simulink model "smc"  (R2018a)
settings: Solver=VariableStepAuto  StartTime=0.0  StopTime=500  RelTol=1e-3
values from neighbouring files (symbols this model uses):
  D = 0    [k_func.m]
libraries: simulink_extras x5, dspmtrx3 x3, sharedutil x3
settings Model: Creator=Renz  LastModifiedBy=Renz

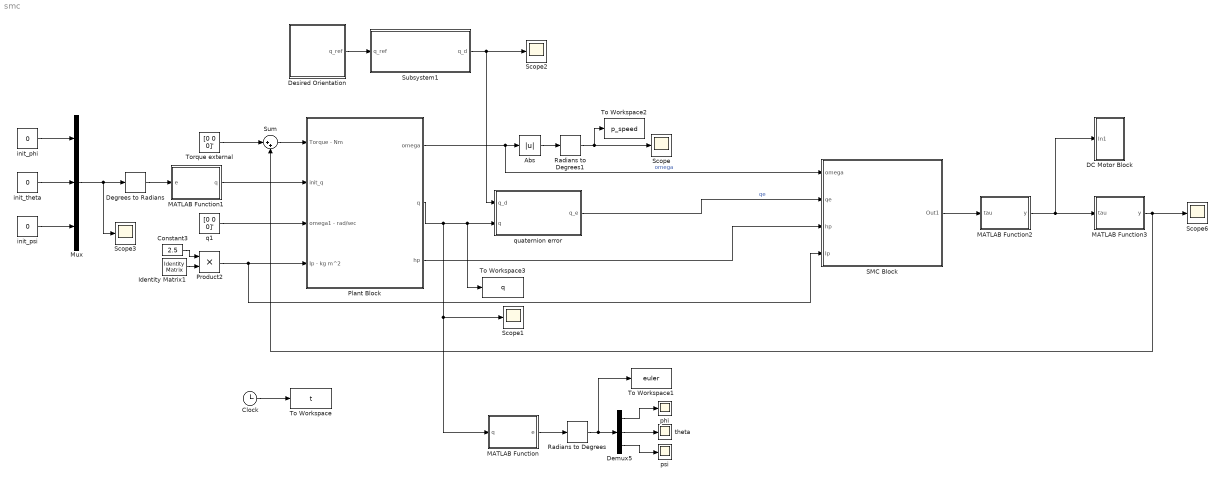
== system smc ==
  Abs : Abs
  Clock : Clock
  Constant3 : Constant  Value=2.5
  DC Motor Block : Subsystem
  Degrees to Radians : simulink_extras/Transformations/Degrees to Radians
  Demux5 : Demux  Outputs=3
  Desired Orientation : Subsystem
  Identity Matrix1 : dspmtrx3/Identity Matrix  Inherit=off  N=3  Ts=1  dataType=double  isSigned=on  wordLen=16  udDataType=sfix(16)  fracBitsMode=Best precision  numFracBits=15  OutDataTypeStr=double  LastOutDataTypeStr=double
      settings: SourceProductName=DSP System Toolbox
  MATLAB Function : MATLAB Function  TreatAsAtomicUnit=on
  MATLAB Function1 : MATLAB Function  TreatAsAtomicUnit=on
  MATLAB Function2 : MATLAB Function  TreatAsAtomicUnit=on
  MATLAB Function3 : MATLAB Function  TreatAsAtomicUnit=on
  Mux : Mux  Inputs=3
  Plant Block : Subsystem
  Product2 : Product
  Radians to Degrees : simulink_extras/Transformations/Radians to Degrees
  Radians to Degrees1 : simulink_extras/Transformations/Radians to Degrees
  SMC Block : Subsystem
  Scope{,1..3,6} (5 alike) : Scope
  Subsystem1 : Subsystem
  Sum : Sum  Inputs=|++
  To Workspace : ToWorkspace  VariableName=t  SampleTime=-1
  To Workspace1 : ToWorkspace  VariableName=euler  SampleTime=-1
  To Workspace2 : ToWorkspace  VariableName=p_speed  SampleTime=-1
  To Workspace3 : ToWorkspace  VariableName=q  SampleTime=-1
  Torque external : Constant  Value=[0 0 0]'
  init_phi : Constant  Value=0
  init_psi : Constant  Value=0
  init_theta : Constant  Value=0
  phi : Scope
  psi : Scope
  q1 : Constant  Value=[0 0 0]'
  quaternion error : Subsystem
  theta : Scope
  wires:
  Identity Matrix1/1 -> Product2/2
  MATLAB Function1/1(q) -> Plant Block/2(init_q)
  Torque external/1 -> Sum/1
  init_psi/1 -> Mux/3
  MATLAB Function2/1(y) -> DC Motor Block/1(In1), MATLAB Function3/1(tau)
  Demux5/1 -> phi/1
  Mux/1 -> Scope3/1, Degrees to Radians/1
  Demux5/3 -> psi/1
  Clock/1 -> To Workspace/1
  Plant Block/2(q) -> MATLAB Function/1(q), Scope1/1, To Workspace3/1, quaternion error/2(q)
  Demux5/2 -> theta/1
  Desired Orientation/1(q_ref) -> Subsystem1/1(q_ref)
  Radians to Degrees/1 -> To Workspace1/1, Demux5/1
  Degrees to Radians/1 -> MATLAB Function1/1(e)
  Product2/1 -> SMC Block/4(Ip), Plant Block/4(Ip - kg m^2)
  MATLAB Function/1(e) -> Radians to Degrees/1
  Constant3/1 -> Product2/1
  Sum/1 -> Plant Block/1(Torque - Nm)
  init_theta/1 -> Mux/2
  Plant Block/1(omega) -> SMC Block/1(omega), Abs/1  "omega"
  Subsystem1/1(q_d) -> Scope2/1, quaternion error/1(q_d)
  init_phi/1 -> Mux/1
  q1/1 -> Plant Block/3(omega1 - rad/sec)
  Abs/1 -> Radians to Degrees1/1
  Radians to Degrees1/1 -> Scope/1, To Workspace2/1
  MATLAB Function3/1(y) -> Scope6/1, Sum/2
  quaternion error/1(q_e) -> SMC Block/2(qe)  "qe"
  Plant Block/3(hp) -> SMC Block/3(hp)
  SMC Block/1(Out1) -> MATLAB Function2/1(tau)

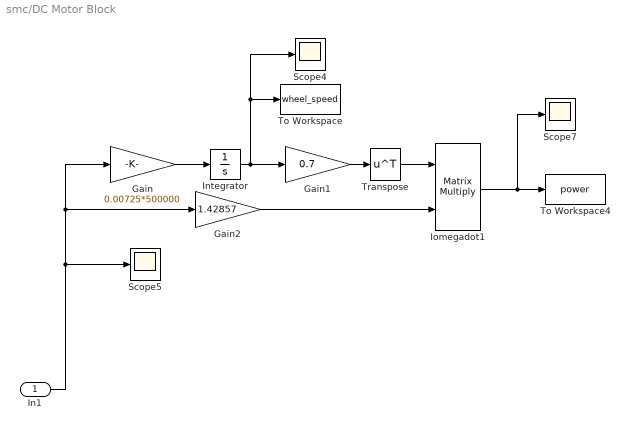
== system smc/DC Motor Block ==
  In1 : Inport
  Gain : Gain  Gain=0.00725*500000
  Gain1 : Gain  Gain=0.7
  Gain2 : Gain  Gain=1.42857
  Integrator : Integrator
  Iomegadot1 : Product  Multiplication=Matrix(*)
  Scope4 : Scope
  Scope5 : Scope
  Scope7 : Scope
  To Workspace : ToWorkspace  VariableName=wheel_speed  SampleTime=-1
  To Workspace4 : ToWorkspace  VariableName=power  SampleTime=-1
  Transpose : Math  Operator=transpose  SaturateOnIntegerOverflow=on
  wires:
  Gain/1 -> Integrator/1
  Gain2/1 -> Iomegadot1/2
  Iomegadot1/1 -> Scope7/1, To Workspace4/1
  Transpose/1 -> Iomegadot1/1
  In1/1 -> Scope5/1, Gain2/1, Gain/1
  Integrator/1 -> Scope4/1, To Workspace/1, Gain1/1
  Gain1/1 -> Transpose/1

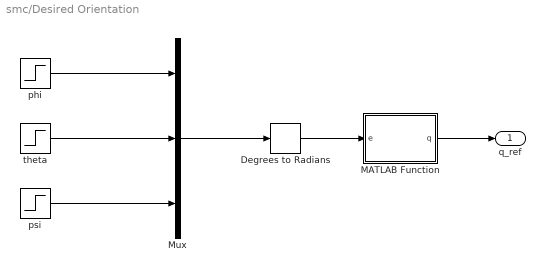
== system smc/Desired Orientation ==
  Degrees to Radians : simulink_extras/Transformations/Degrees to Radians
  MATLAB Function : MATLAB Function  TreatAsAtomicUnit=on
  Mux : Mux  Inputs=3
  phi : Step  After=80  SampleTime=0
  psi : Step  After=60  SampleTime=0
  theta : Step  After=40  SampleTime=0
  q_ref : Outport
  wires:
  Mux/1 -> Degrees to Radians/1
  psi/1 -> Mux/3
  phi/1 -> Mux/1
  theta/1 -> Mux/2
  MATLAB Function/1(q) -> q_ref/1
  Degrees to Radians/1 -> MATLAB Function/1(e)

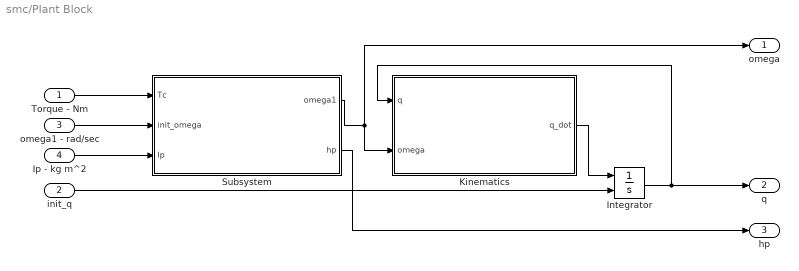
== system smc/Plant Block ==
  Torque - Nm : Inport
  init_q : Inport  Port=2
  omega1 - rad/sec : Inport  Port=3
  Ip - kg m^2 : Inport  Port=4
  Integrator : Integrator  InitialConditionSource=external
  Kinematics : Subsystem
  Subsystem : Subsystem
  omega : Outport
  q : Outport  Port=2
  hp : Outport  Port=3
  wires:
  Kinematics/1(q_dot) -> Integrator/1
  Integrator/1 -> Kinematics/1(q), q/1
  Torque - Nm/1 -> Subsystem/1(Tc)
  omega1 - rad/sec/1 -> Subsystem/2(init_omega)
  init_q/1 -> Integrator/2
  Subsystem/1(omega1) -> Kinematics/2(omega), omega/1
  Ip - kg m^2/1 -> Subsystem/3(Ip)
  Subsystem/2(hp) -> hp/1

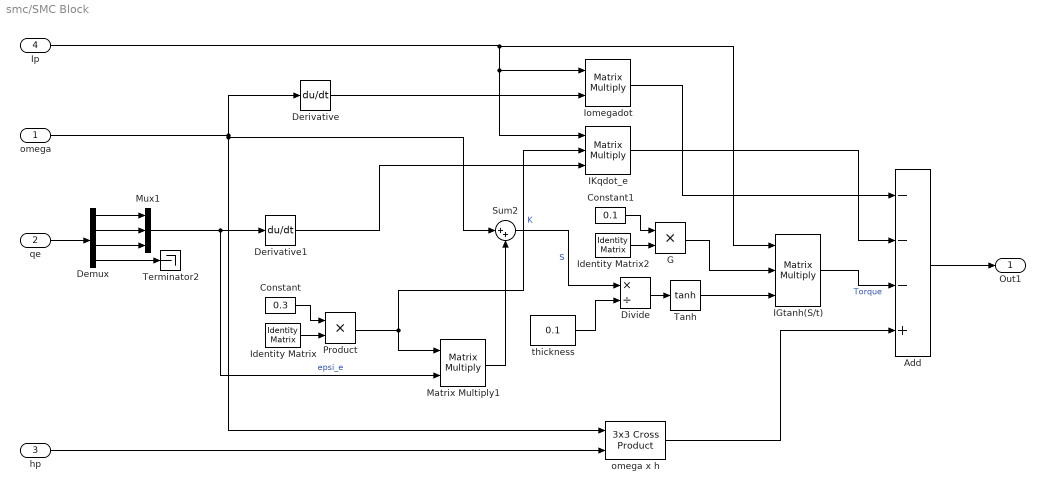
== system smc/SMC Block ==
  omega : Inport
  qe : Inport  Port=2
  hp : Inport  Port=3
  Ip : Inport  Port=4
  Add : Sum  Inputs=---+
  Constant : Constant  Value=0.3
  Constant1 : Constant  Value=0.1
  Demux : Demux
  Derivative : Derivative
  Derivative1 : Derivative
  Divide : Product  Inputs=*/
  G : Product
  IGtanh(S/t) : Product  Inputs=3  Multiplication=Matrix(*)
  IKqdot_e : Product  Inputs=3  Multiplication=Matrix(*)
  Identity Matrix : dspmtrx3/Identity Matrix  Inherit=off  N=3  Ts=1  dataType=double  isSigned=on  wordLen=16  udDataType=sfix(16)  fracBitsMode=Best precision  numFracBits=15  OutDataTypeStr=double  LastOutDataTypeStr=double
      settings: SourceProductName=DSP System Toolbox
  Identity Matrix2 : dspmtrx3/Identity Matrix  Inherit=off  N=3  Ts=1  dataType=double  isSigned=on  wordLen=16  udDataType=sfix(16)  fracBitsMode=Best precision  numFracBits=15  OutDataTypeStr=double  LastOutDataTypeStr=double
      settings: SourceProductName=DSP System Toolbox
  Iomegadot : Product  Multiplication=Matrix(*)
  Matrix Multiply1 : Product  Multiplication=Matrix(*)
  Mux1 : Mux  Inputs=3
  Product : Product
  Sum2 : Sum  Inputs=|++
  Tanh : Trigonometry  Operator=tanh
  Terminator2 : Terminator
  omega x h : sharedutil/3x3 Cross Product  aMode=aMode
      settings: SourceProductBaseCode=AE
  thickness : Constant  Value=0.1
  Out1 : Outport
  wires:
  Divide/1 -> Tanh/1
  Derivative1/1 -> IKqdot_e/3
  IGtanh(S/t)/1 -> Add/3  "Torque"
  Ip/1 -> IKqdot_e/1, Iomegadot/1, IGtanh(S/t)/1
  Derivative/1 -> Iomegadot/2
  Add/1 -> Out1/1
  omega/1 -> omega x h/1, Sum2/1, Derivative/1
  Product/1 -> IKqdot_e/2, Matrix Multiply1/1  "K"
  Tanh/1 -> IGtanh(S/t)/3
  Matrix Multiply1/1 -> Sum2/2
  Identity Matrix/1 -> Product/2
  thickness/1 -> Divide/2
  G/1 -> IGtanh(S/t)/2
  omega x h/1 -> Add/4
  Constant/1 -> Product/1
  Constant1/1 -> G/1
  Mux1/1 -> Matrix Multiply1/2, Derivative1/1  "epsi_e"
  IKqdot_e/1 -> Add/2
  Sum2/1 -> Divide/1  "S"
  hp/1 -> omega x h/2
  Iomegadot/1 -> Add/1
  Identity Matrix2/1 -> G/2
  Demux/1 -> Mux1/1
  qe/1 -> Demux/1
  Demux/2 -> Mux1/2
  Demux/3 -> Mux1/3
  Demux/4 -> Terminator2/1

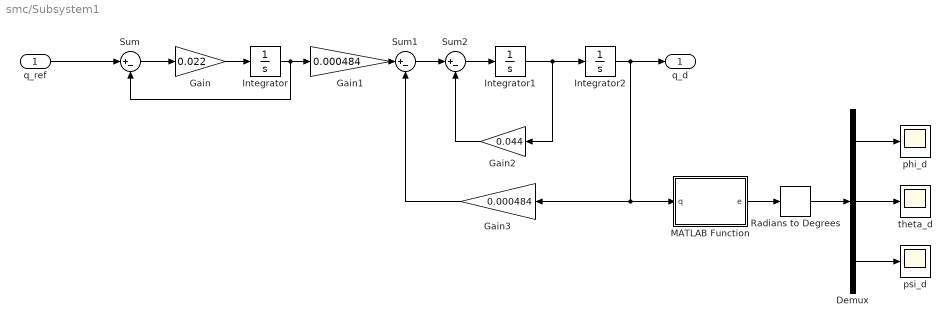
== system smc/Subsystem1 ==
  q_ref : Inport
  Demux : Demux  Outputs=3
  Gain : Gain  Gain=0.022
  Gain1 : Gain  Gain=0.000484
  Gain2 : Gain  Gain=0.044
  Gain3 : Gain  Gain=0.000484
  Integrator : Integrator
  Integrator1 : Integrator
  Integrator2 : Integrator
  MATLAB Function : MATLAB Function  TreatAsAtomicUnit=on
  Radians to Degrees : simulink_extras/Transformations/Radians to Degrees
  Sum : Sum  Inputs=|+-
  Sum1 : Sum  Inputs=|+-
  Sum2 : Sum  Inputs=|+-
  phi_d : Scope
  psi_d : Scope
  theta_d : Scope
  q_d : Outport
  wires:
  Demux/3 -> psi_d/1
  Gain1/1 -> Sum1/1
  Sum/1 -> Gain/1
  Gain2/1 -> Sum2/2
  Demux/2 -> theta_d/1
  Gain/1 -> Integrator/1
  Integrator/1 -> Gain1/1, Sum/2
  Sum1/1 -> Sum2/1
  Gain3/1 -> Sum1/2
  Integrator1/1 -> Gain2/1, Integrator2/1
  Sum2/1 -> Integrator1/1
  q_ref/1 -> Sum/1
  Demux/1 -> phi_d/1
  Radians to Degrees/1 -> Demux/1
  Integrator2/1 -> q_d/1, MATLAB Function/1(q), Gain3/1
  MATLAB Function/1(e) -> Radians to Degrees/1

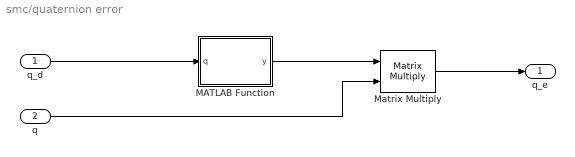
== system smc/quaternion error ==
  q_d : Inport
  q : Inport  Port=2
  MATLAB Function : MATLAB Function  TreatAsAtomicUnit=on
  Matrix Multiply : Product  Multiplication=Matrix(*)
  q_e : Outport
  wires:
  MATLAB Function/1(y) -> Matrix Multiply/1
  Matrix Multiply/1 -> q_e/1
  q/1 -> Matrix Multiply/2
  q_d/1 -> MATLAB Function/1(q)

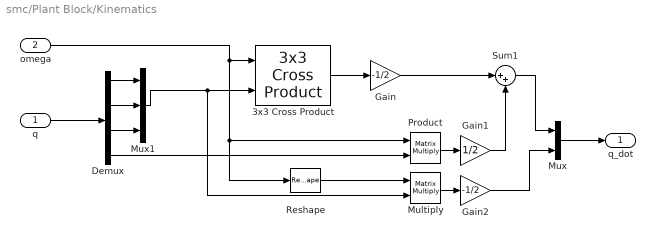
== system smc/Plant Block/Kinematics ==
  q : Inport
  omega : Inport  Port=2
  3x3 Cross Product : sharedutil/3x3 Cross Product  aMode=aMode
      settings: SourceProductBaseCode=AE
  Demux : Demux
  Gain : Gain  Gain=-1/2
  Gain1 : Gain  Gain=1/2
  Gain2 : Gain  Gain=-1/2
  Multiply : Product  Multiplication=Matrix(*)
  Mux : Mux  Inputs=2
  Mux1 : Mux  Inputs=3
  Product : Product  Multiplication=Matrix(*)
  Reshape : Reshape  OutputDimensionality=Row vector (2-D)
  Sum1 : Sum  Inputs=|++
  q_dot : Outport
  wires:
  omega/1 -> 3x3 Cross Product/1, Product/1, Reshape/1
  q/1 -> Demux/1
  Mux1/1 -> Multiply/2, 3x3 Cross Product/2
  Gain1/1 -> Sum1/2
  3x3 Cross Product/1 -> Gain/1
  Product/1 -> Gain1/1
  Multiply/1 -> Gain2/1
  Gain/1 -> Sum1/1
  Demux/4 -> Product/2
  Reshape/1 -> Multiply/1
  Mux/1 -> q_dot/1
  Sum1/1 -> Mux/1
  Gain2/1 -> Mux/2
  Demux/2 -> Mux1/2
  Demux/1 -> Mux1/1
  Demux/3 -> Mux1/3

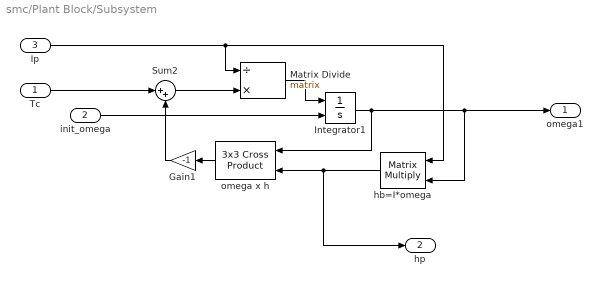
== system smc/Plant Block/Subsystem ==
  Tc : Inport
  init_omega : Inport  Port=2
  Ip : Inport  Port=3
  Gain1 : Gain  Gain=-1
  Integrator1 : Integrator  InitialConditionSource=external  ZeroCross=off
  Matrix Divide : Product  Inputs=/*  Multiplication=Matrix(*)
  Sum2 : Sum  Inputs=|++
  hb=I*omega : Product  Multiplication=Matrix(*)
  omega x h : sharedutil/3x3 Cross Product  aMode=aMode
      settings: SourceProductBaseCode=AE
  omega1 : Outport
  hp : Outport  Port=2
  wires:
  Gain1/1 -> Sum2/2
  Integrator1/1 -> omega x h/1, omega1/1, hb=I*omega/2
  init_omega/1 -> Integrator1/2
  Sum2/1 -> Matrix Divide/2
  hb=I*omega/1 -> hp/1, omega x h/2
  omega x h/1 -> Gain1/1
  Tc/1 -> Sum2/1
  Matrix Divide/1 -> Integrator1/1
  Ip/1 -> Matrix Divide/1, hb=I*omega/1

== matlab function smc/Subsystem1/MATLAB Function ==
  data: q input; e output
function e = quat2euler(q)

q0 = q(1,:);
q1 = q(2,:);
q2 = q(3,:);
q3 = q(4,:);

phi = atan((2*(q2*q3 + q0*q1))/(q0^2 - q1^2 - q2^2 + q3^2)); 
theta = asin(-2*(q1*q3 - q0*q2));
psi = atan((2*(q1*q2 + q0*q3))/(q0^2 + q1^2 -q2^2 - q3^2)); 

e = [phi;theta;psi];

end

== matlab function smc/Desired Orientation/MATLAB Function ==
  data: e input; q output
function q = euler2quat(e)

e1 = 0.5*e(1,:);
e2 = 0.5*e(2,:);
e3 = 0.5*e(3,:);

q0 = (sin(e1)*sin(e2)*sin(e3)) + (cos(e1)*cos(e2)*cos(e3));
q1 = (-sin(e2)*sin(e3)*cos(e1)) + (sin(e1)*cos(e2)*cos(e3));
q2 = (sin(e1)*cos(e2)*sin(e3)) + (sin(e2)*cos(e1)*cos(e3));
q3 = (sin(e3)*cos(e1)*cos(e2)) - (sin(e1)*sin(e2)*cos(e3));

q = [q0;q1;q2;q3];

end

== matlab function smc/MATLAB Function1 ==
  data: e input; q output
function q = euler2quat(e)

e1 = 0.5*e(1,:);
e2 = 0.5*e(2,:);
e3 = 0.5*e(3,:);

q0 = (sin(e1)*sin(e2)*sin(e3)) + (cos(e1)*cos(e2)*cos(e3));
q1 = (-sin(e2)*sin(e3)*cos(e1)) + (sin(e1)*cos(e2)*cos(e3));
q2 = (sin(e1)*cos(e2)*sin(e3)) + (sin(e2)*cos(e1)*cos(e3));
q3 = (sin(e3)*cos(e1)*cos(e2)) - (sin(e1)*sin(e2)*cos(e3));

q = [q0;q1;q2;q3];

end

== matlab function smc/MATLAB Function3 ==
  data: tau input; y output
function y = torque(tau)
L = [0.57735, -0.57735, -0.57735, 0.57735; 0.57735, -0.57735, 0.57735, -0.57735; 0.57735, 0.57735, -0.57735, -0.57735];


y = L*tau;

== matlab function smc/quaternion error/MATLAB Function ==
  data: q input; y output
function y = q_error(q)
q1 = q(1,:);
q2 = q(2,:);
q3 = q(3,:);
q4 = q(4,:);

y = [q4,q3,-q2,-q1; -q3,q4,q1,-q2; q2,-q1,q4,-q3; q1,q2,q3,q4];

== matlab function smc/MATLAB Function ==
  data: q input; e output
function e = quat2euler(q)

q0 = q(1,:);
q1 = q(2,:);
q2 = q(3,:);
q3 = q(4,:);

phi = atan((2*(q2*q3 + q0*q1))/(q0^2 - q1^2 - q2^2 + q3^2)); 
theta = asin(-2*(q1*q3 - q0*q2));
psi = atan((2*(q1*q2 + q0*q3))/(q0^2 + q1^2 -q2^2 - q3^2)); 

e = [phi;theta;psi];

end

== matlab function smc/MATLAB Function2 ==
  data: tau input; y output
function y = control_alloc(tau)
K =[1 0 0 0 
    0 1 0 0 
    0 0 1 0 
    0 0 0 1];
T = [0.57735, -0.57735, -0.57735, 0.57735; 0.57735, -0.57735, 0.57735, -0.57735; 0.57735, 0.57735, -0.57735, -0.57735];
W = [1 0 0 0     
    0 1 0 0      
    0 0 1 0      
    0 0 0 1];


y = ucalloc(K,T,W,tau);
